simulink subsystem "VehicleDynamicsRing_subsysref"  (R2020a)
settings: Solver=VariableStepAuto  StartTime=0.0  StopTime=10.0  RelTol=1e-3
undefined symbols (not defined in the file): DRIVE_MODE, VDR
settings Model: Creator=Kiera  LastModifiedBy=Kiera

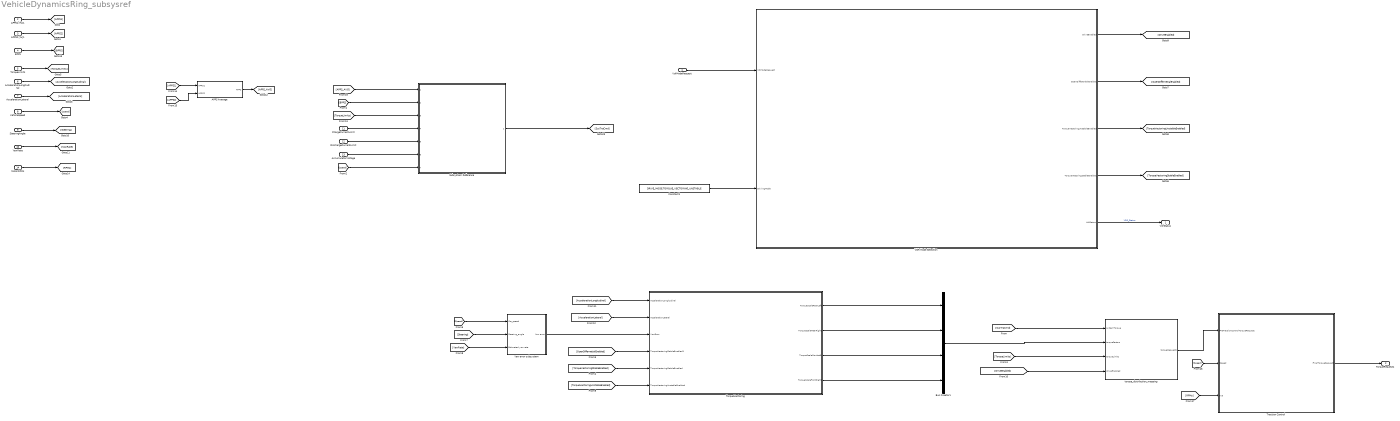
== system VehicleDynamicsRing_subsysref ==
  VdrModeRequest : Inport  OutDataTypeStr=Enum: MSR_REQUEST
  APPS1 [%]1 : Inport  Port=2  OutDataTypeStr=double
  APPS2 [%]1 : Inport  Port=3  OutDataTypeStr=double
  BPPS : Inport  Port=4  OutDataTypeStr=double
  TorqueLimits : Inport  Port=5  OutDataTypeStr=Bus: TorqueLimits
  AccelerationLongitudinal : Inport  Port=6  OutDataTypeStr=double
  AccelerationLateral : Inport  Port=7  OutDataTypeStr=double
  VehicleSpeed : Inport  Port=8
  SteeringAngle : Inport  Port=9
  YawRate : Inport  Port=10
  ChargeCurrentLimit : Inport  Port=11  OutDataTypeStr=double
  DischargeCurrentLimit : Inport  Port=12  OutDataTypeStr=double
  AccumulatorVoltage : Inport  Port=13
  MotorRPMs : Inport  Port=14  OutDataTypeStr=Bus: MotorRPMs
  APPS Average : Subsystem
  Bus Creator1 : BusCreator  Inputs=4
  Constant1 : Constant  Value=DRIVE_MODE.TORQUE_VECTORING_UNSTABLE
  Subsystem Reference : Subsystem  ReferencedSubsystem=PedalMapping_subsysref
  TorqueVectoring : Subsystem
  Traction Control : Subsystem
  VDR Mode Selection : Stateflow chart  TreatAsAtomicUnit=on
  Yaw error subsystem : Subsystem
  torque_distribution_mapping : MATLAB Function  TreatAsAtomicUnit=on
  VdrStatus : Outport  OutDataTypeStr=Enum: RING_STATUS  VectorParamsAs1DForOutWhenUnconnected=off
  TorqueRequests : Outport  Port=2  OutDataTypeStr=Bus: TorqueRequests  VectorParamsAs1DForOutWhenUnconnected=off
  wires:
  Yaw error subsystem/1(Yaw error) -> TorqueVectoring/3(YawError)
  YawRate/1 -> [YawRate]
  APPS2 [%]1/1 -> [APPS2]
  APPS1 [%]1/1 -> [APPS1]
  Bus Creator1/1 -> torque_distribution_mapping/2(torqueFactors)
  [OpenDiffernetialEnabled] -> TorqueVectoring/4(TorqueVectoringStableEnabled1)
  [Speed] -> Traction Control/2(Speed)
  MotorRPMs/1 -> [RPMs]
  TorqueVectoring/4(TorqueScaleFrontRight) -> Bus Creator1/4
  [RPMs] -> Traction Control/3(In3)
  Traction Control/1(FinalTorqueRequest) -> TorqueRequests/1
  VDR Mode Selection/3(TorqueVectoringUnstableEnabled) -> [TorqueVectoringUnstableEnabled]
  TorqueVectoring/3(TorqueScaleFrontLeft) -> Bus Creator1/3
  AccumulatorVoltage/1 -> Subsystem Reference/6
  [APPS2] -> APPS Average/2(APPS2)
  torque_distribution_mapping/1(torqueRequests) -> Traction Control/1(PreTractionControlTorqueRequest)
  VdrModeRequest/1 -> VDR Mode Selection/1(VdrModeRequest)
  DischargeCurrentLimit/1 -> Subsystem Reference/5
  BPPS/1 -> [BPPS]
  APPS Average/1(APPS) -> [APPS_AVG]
  VehicleSpeed/1 -> [Speed]
  Subsystem Reference/1 -> [SysTrqCmd]
  [SysTrqCmd] -> torque_distribution_mapping/1(systemTorque)
  AccelerationLongitudinal/1 -> [AccelerationLongitudinal]
  [APPS_AVG] -> Subsystem Reference/1
  [APPS1] -> APPS Average/1(APPS1)
  [Speed] -> Yaw error subsystem/1(Car_speed)
  TorqueVectoring/1(TorqueScaleRearLeft) -> Bus Creator1/1
  [YawRate] -> Yaw error subsystem/3("Estimated yaw rate ")
  [TorqueLimits] -> torque_distribution_mapping/3(torqueLimits)
  SteeringAngle/1 -> [Steering]
  Constant1/1 -> VDR Mode Selection/2(DrivingMode)
  [DriveEnabled] -> torque_distribution_mapping/4(driveEnabled)
  [AccelerationLongitudinal] -> TorqueVectoring/1("AccelerationLongitudinal ")
  VDR Mode Selection/1(DriveEnabled) -> [DriveEnabled]
  AccelerationLateral/1 -> [AccelerationLateral]
  VDR Mode Selection/5(VdrStatus) -> VdrStatus/1  "VDR_Status"
  [TorqueVectoringUnstableEnabled] -> TorqueVectoring/6(TorqueVectoringUnstableEnabled)
  [TorqueLimits] -> Subsystem Reference/3
  [BPPS] -> Subsystem Reference/2
  VDR Mode Selection/2(OpenDifferentialEnabled) -> [OpenDiffernetialEnabled]
  TorqueLimits/1 -> [TorqueLimits]
  [TorqueVectoringStableEnabled] -> TorqueVectoring/5(TorqueVectoringStableEnabled)
  [Steering] -> Yaw error subsystem/2(Steering_angle)
  ChargeCurrentLimit/1 -> Subsystem Reference/4
  [Speed] -> Subsystem Reference/7
  VDR Mode Selection/4(TorqueVectoringStableEnabled) -> [TorqueVectoringStableEnabled]
  [AccelerationLateral] -> TorqueVectoring/2(AccelerationLateral)
  TorqueVectoring/2(TorqueScaleRearRight) -> Bus Creator1/2

== system VehicleDynamicsRing_subsysref/APPS Average ==
  APPS1 : Inport
  APPS2 : Inport  Port=2
  Add : Sum
  Constant : Constant  Value=2
  Divide : Product  Inputs=*/
  APPS : Outport  VectorParamsAs1DForOutWhenUnconnected=off
  wires:
  Divide/1 -> APPS/1
  APPS2/1 -> Add/2
  APPS1/1 -> Add/1
  Add/1 -> Divide/1
  Constant/1 -> Divide/2

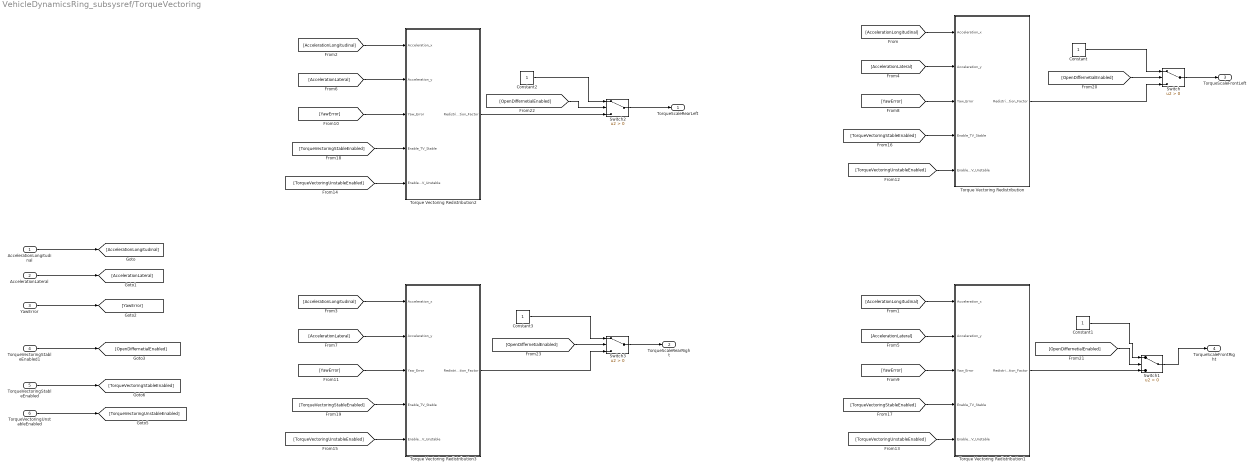
== system VehicleDynamicsRing_subsysref/TorqueVectoring ==
  "AccelerationLongitudinal " : Inport
  AccelerationLateral : Inport  Port=2
  YawError : Inport  Port=3
  TorqueVectoringStableEnabled1 : Inport  Port=4
  TorqueVectoringStableEnabled : Inport  Port=5
  TorqueVectoringUnstableEnabled : Inport  Port=6
  Constant{,1..3} (4 alike) : Constant
  Switch{,1..3} (4 alike) : Switch  Criteria=u2 > Threshold
  Torque Vectoring Redistribution : Subsystem  AncestorBlock=TorqueVectoringAlgorithmLib/Torque Vectoring Redistribution  mask{wheel_1=Front, wheel_2=Left}
      mask prompts: wheel_1 "Front or Rear Wheel"; wheel_2 "Left or Right Wheel"
      mask init:
      | %Front vs Rear Modifier
      | if(wheel_1 == 1) %Front Wheel
      |     stable_longitudinal_mod = -1;
      | else %Rear Wheel
      |     stable_longitudinal_mod = 1;
      | end
      | 
      | %Left vs Rear Modifier
      | if(wheel_2 == 1) %Left Wheel
      |     unstable_mod = -1;
      |     stable_lateral_mod = -1;
      | else %Right Wheel
      |     unstable_mod = 1;
      |     stable_lateral_mod = 1;
      | end
      mask TypeOptions wheel_1: Front | Rear
      mask TypeOptions wheel_2: Left | Right
      mask DialogControl DescGroupVar Prompt: Torque Vectoring Configurations
      mask DialogControl DescTextVar Prompt: Select the wheel for the torque vectoring configuration.
  Torque Vectoring Redistribution1 : Subsystem  AncestorBlock=TorqueVectoringAlgorithmLib/Torque Vectoring Redistribution  mask{wheel_1=Front, wheel_2=Right}
      mask prompts: wheel_1 "Front or Rear Wheel"; wheel_2 "Left or Right Wheel"
      mask init: same as VehicleDynamicsRing_subsysref/TorqueVectoring/Torque Vectoring Redistribution
      mask TypeOptions wheel_1: Front | Rear
      mask TypeOptions wheel_2: Left | Right
      mask DialogControl DescGroupVar Prompt: Torque Vectoring Configurations
      mask DialogControl DescTextVar Prompt: Select the wheel for the torque vectoring configuration.
  Torque Vectoring Redistribution2 : Subsystem  AncestorBlock=TorqueVectoringAlgorithmLib/Torque Vectoring Redistribution  mask{wheel_1=Rear, wheel_2=Left}
      mask prompts: wheel_1 "Front or Rear Wheel"; wheel_2 "Left or Right Wheel"
      mask init: same as VehicleDynamicsRing_subsysref/TorqueVectoring/Torque Vectoring Redistribution
      mask TypeOptions wheel_1: Front | Rear
      mask TypeOptions wheel_2: Left | Right
      mask DialogControl DescGroupVar Prompt: Torque Vectoring Configurations
      mask DialogControl DescTextVar Prompt: Select the wheel for the torque vectoring configuration.
  Torque Vectoring Redistribution3 : Subsystem  AncestorBlock=TorqueVectoringAlgorithmLib/Torque Vectoring Redistribution  mask{wheel_1=Rear, wheel_2=Right}
      mask prompts: wheel_1 "Front or Rear Wheel"; wheel_2 "Left or Right Wheel"
      mask init: same as VehicleDynamicsRing_subsysref/TorqueVectoring/Torque Vectoring Redistribution
      mask TypeOptions wheel_1: Front | Rear
      mask TypeOptions wheel_2: Left | Right
      mask DialogControl DescGroupVar Prompt: Torque Vectoring Configurations
      mask DialogControl DescTextVar Prompt: Select the wheel for the torque vectoring configuration.
  TorqueScaleRearLeft : Outport  VectorParamsAs1DForOutWhenUnconnected=off
  TorqueScaleRearRight : Outport  Port=2  VectorParamsAs1DForOutWhenUnconnected=off
  TorqueScaleFrontLeft : Outport  Port=3  VectorParamsAs1DForOutWhenUnconnected=off
  TorqueScaleFrontRight : Outport  Port=4  VectorParamsAs1DForOutWhenUnconnected=off
  wires:
  "AccelerationLongitudinal "/1 -> [AccelerationLongitudinal]
  AccelerationLateral/1 -> [AccelerationLateral]
  YawError/1 -> [YawError]
  TorqueVectoringUnstableEnabled/1 -> [TorqueVectoringUnstableEnabled]
  [AccelerationLongitudinal] -> Torque Vectoring Redistribution2/1(Acceleration_x)
  [AccelerationLongitudinal] -> Torque Vectoring Redistribution3/1(Acceleration_x)
  [AccelerationLateral] -> Torque Vectoring Redistribution2/2(Acceleration_y)
  [AccelerationLateral] -> Torque Vectoring Redistribution3/2(Acceleration_y)
  [YawError] -> Torque Vectoring Redistribution2/3(Yaw_Error)
  [YawError] -> Torque Vectoring Redistribution3/3(Yaw_Error)
  TorqueVectoringStableEnabled/1 -> [TorqueVectoringStableEnabled]
  [TorqueVectoringUnstableEnabled] -> Torque Vectoring Redistribution2/5(Enable_TV_Unstable)
  [TorqueVectoringUnstableEnabled] -> Torque Vectoring Redistribution3/5(Enable_TV_Unstable)
  [TorqueVectoringStableEnabled] -> Torque Vectoring Redistribution2/4(Enable_TV_Stable)
  [TorqueVectoringStableEnabled] -> Torque Vectoring Redistribution3/4(Enable_TV_Stable)
  TorqueVectoringStableEnabled1/1 -> [OpenDiffernetialEnabled]
  [TorqueVectoringStableEnabled] -> Torque Vectoring Redistribution/4(Enable_TV_Stable)
  [TorqueVectoringUnstableEnabled] -> Torque Vectoring Redistribution/5(Enable_TV_Unstable)
  [YawError] -> Torque Vectoring Redistribution/3(Yaw_Error)
  [AccelerationLateral] -> Torque Vectoring Redistribution/2(Acceleration_y)
  [AccelerationLongitudinal] -> Torque Vectoring Redistribution/1(Acceleration_x)
  [TorqueVectoringStableEnabled] -> Torque Vectoring Redistribution1/4(Enable_TV_Stable)
  [YawError] -> Torque Vectoring Redistribution1/3(Yaw_Error)
  [AccelerationLongitudinal] -> Torque Vectoring Redistribution1/1(Acceleration_x)
  [TorqueVectoringUnstableEnabled] -> Torque Vectoring Redistribution1/5(Enable_TV_Unstable)
  [AccelerationLateral] -> Torque Vectoring Redistribution1/2(Acceleration_y)
  [OpenDiffernetialEnabled] -> Switch/2
  Switch/1 -> TorqueScaleFrontLeft/1
  [OpenDiffernetialEnabled] -> Switch1/2
  Switch1/1 -> TorqueScaleFrontRight/1
  Constant1/1 -> Switch1/1
  Torque Vectoring Redistribution1/1(Redistribution_Factor) -> Switch1/3
  Torque Vectoring Redistribution/1(Redistribution_Factor) -> Switch/3
  Constant/1 -> Switch/1
  Constant2/1 -> Switch2/1
  [OpenDiffernetialEnabled] -> Switch2/2
  Switch2/1 -> TorqueScaleRearLeft/1
  Torque Vectoring Redistribution2/1(Redistribution_Factor) -> Switch2/3
  Constant3/1 -> Switch3/1
  [OpenDiffernetialEnabled] -> Switch3/2
  Switch3/1 -> TorqueScaleRearRight/1
  Torque Vectoring Redistribution3/1(Redistribution_Factor) -> Switch3/3

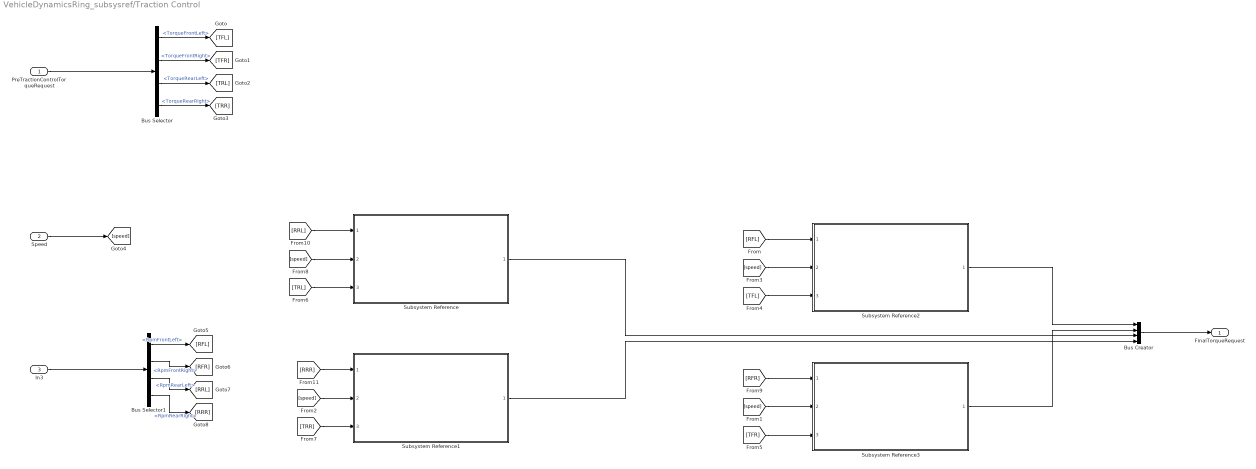
== system VehicleDynamicsRing_subsysref/Traction Control ==
  PreTractionControlTorqueRequest : Inport
  Speed : Inport  Port=2
  In3 : Inport  Port=3
  Bus Creator : BusCreator  Inputs=4  OutDataTypeStr=Bus: TorqueRequests
  Bus Selector : BusSelector  OutputSignals=TorqueFrontLeft,TorqueFrontRight,TorqueRearLeft,TorqueRearRight
  Bus Selector1 : BusSelector  OutputSignals=RpmFrontLeft,RpmFrontRight,RpmRearLeft,RpmRearRight
  Subsystem Reference{,1..3} (4 alike) : Subsystem  ReferencedSubsystem=TractionControl_subsysref
  FinalTorqueRequest : Outport  VectorParamsAs1DForOutWhenUnconnected=off
  wires:
  Subsystem Reference1/1 -> Bus Creator/4
  Subsystem Reference/1 -> Bus Creator/3
  Subsystem Reference3/1 -> Bus Creator/2
  Subsystem Reference2/1 -> Bus Creator/1
  Bus Creator/1 -> FinalTorqueRequest/1
  [RFR] -> Subsystem Reference3/1
  [RFL] -> Subsystem Reference2/1
  [RRL] -> Subsystem Reference/1
  [RRR] -> Subsystem Reference1/1
  Bus Selector1/4 -> [RRR]  "<RpmRearRight>"
  Bus Selector1/3 -> [RRL]  "<RpmRearLeft>"
  Bus Selector1/2 -> [RFR]  "<RpmFrontRight>"
  Bus Selector1/1 -> [RFL]  "<RpmFrontLeft>"
  [speed] -> Subsystem Reference3/2
  [speed] -> Subsystem Reference1/2
  [speed] -> Subsystem Reference2/2
  [speed] -> Subsystem Reference/2
  [TRR] -> Subsystem Reference1/3
  [TRL] -> Subsystem Reference/3
  [TFR] -> Subsystem Reference3/3
  [TFL] -> Subsystem Reference2/3
  In3/1 -> Bus Selector1/1
  Speed/1 -> [speed]
  Bus Selector/4 -> [TRR]  "<TorqueRearRight>"
  Bus Selector/3 -> [TRL]  "<TorqueRearLeft>"
  Bus Selector/2 -> [TFR]  "<TorqueFrontRight>"
  Bus Selector/1 -> [TFL]  "<TorqueFrontLeft>"
  PreTractionControlTorqueRequest/1 -> Bus Selector/1

== system VehicleDynamicsRing_subsysref/Yaw error subsystem ==
  Car_speed : Inport
  Steering_angle : Inport  Port=2
  "Estimated yaw rate " : Inport  Port=3
  Desired yaw rate calculation : Subsystem
  Subtract : Sum  Inputs=+-
  Yaw rate estimatior : Subsystem  Commented=on
  Yaw error : Outport  VectorParamsAs1DForOutWhenUnconnected=off
  wires:
  Steering_angle/1 -> Desired yaw rate calculation/2(Steering angle)
  Subtract/1 -> Yaw error/1
  "Estimated yaw rate "/1 -> Subtract/2
  Car_speed/1 -> Desired yaw rate calculation/1(Car speed)
  Desired yaw rate calculation/1(Desired yaw rate) -> Subtract/1

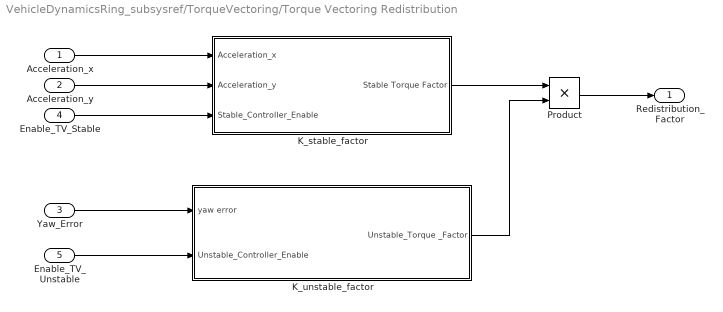
== system VehicleDynamicsRing_subsysref/TorqueVectoring/Torque Vectoring Redistribution ==
  Acceleration_x : Inport
  Acceleration_y : Inport  Port=2
  Yaw_Error : Inport  Port=3
  Enable_TV_Stable : Inport  Port=4
  Enable_TV_Unstable : Inport  Port=5
  K_stable_factor : Subsystem
  K_unstable_factor : Subsystem
  Product : Product
  Redistribution_Factor : Outport  VectorParamsAs1DForOutWhenUnconnected=off
  wires:
  Enable_TV_Unstable/1 -> K_unstable_factor/2(Unstable_Controller_Enable)
  Enable_TV_Stable/1 -> K_stable_factor/3(Stable_Controller_Enable)
  Product/1 -> Redistribution_Factor/1
  Acceleration_y/1 -> K_stable_factor/2(Acceleration_y)
  Yaw_Error/1 -> K_unstable_factor/1(yaw error)
  Acceleration_x/1 -> K_stable_factor/1(Acceleration_x)
  K_stable_factor/1(Stable Torque Factor) -> Product/1
  K_unstable_factor/1(Unstable_Torque _Factor) -> Product/2

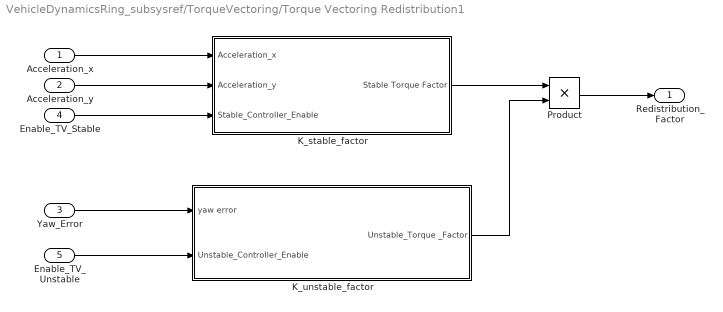
== system VehicleDynamicsRing_subsysref/TorqueVectoring/Torque Vectoring Redistribution1 ==
  Acceleration_x : Inport
  Acceleration_y : Inport  Port=2
  Yaw_Error : Inport  Port=3
  Enable_TV_Stable : Inport  Port=4
  Enable_TV_Unstable : Inport  Port=5
  K_stable_factor : Subsystem
  K_unstable_factor : Subsystem
  Product : Product
  Redistribution_Factor : Outport  VectorParamsAs1DForOutWhenUnconnected=off
  wires:
  Enable_TV_Unstable/1 -> K_unstable_factor/2(Unstable_Controller_Enable)
  Enable_TV_Stable/1 -> K_stable_factor/3(Stable_Controller_Enable)
  Product/1 -> Redistribution_Factor/1
  Acceleration_y/1 -> K_stable_factor/2(Acceleration_y)
  Yaw_Error/1 -> K_unstable_factor/1(yaw error)
  Acceleration_x/1 -> K_stable_factor/1(Acceleration_x)
  K_stable_factor/1(Stable Torque Factor) -> Product/1
  K_unstable_factor/1(Unstable_Torque _Factor) -> Product/2

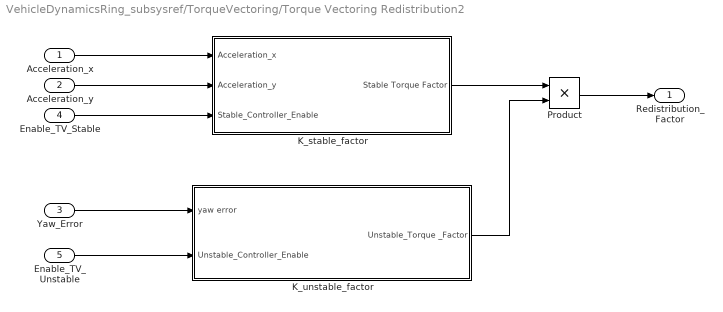
== system VehicleDynamicsRing_subsysref/TorqueVectoring/Torque Vectoring Redistribution2 ==
  Acceleration_x : Inport
  Acceleration_y : Inport  Port=2
  Yaw_Error : Inport  Port=3
  Enable_TV_Stable : Inport  Port=4
  Enable_TV_Unstable : Inport  Port=5
  K_stable_factor : Subsystem
  K_unstable_factor : Subsystem
  Product : Product
  Redistribution_Factor : Outport  VectorParamsAs1DForOutWhenUnconnected=off
  wires:
  Enable_TV_Unstable/1 -> K_unstable_factor/2(Unstable_Controller_Enable)
  Enable_TV_Stable/1 -> K_stable_factor/3(Stable_Controller_Enable)
  Product/1 -> Redistribution_Factor/1
  Acceleration_y/1 -> K_stable_factor/2(Acceleration_y)
  Yaw_Error/1 -> K_unstable_factor/1(yaw error)
  Acceleration_x/1 -> K_stable_factor/1(Acceleration_x)
  K_stable_factor/1(Stable Torque Factor) -> Product/1
  K_unstable_factor/1(Unstable_Torque _Factor) -> Product/2

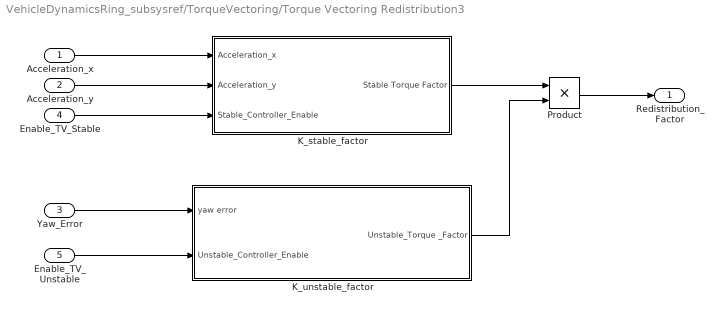
== system VehicleDynamicsRing_subsysref/TorqueVectoring/Torque Vectoring Redistribution3 ==
  Acceleration_x : Inport
  Acceleration_y : Inport  Port=2
  Yaw_Error : Inport  Port=3
  Enable_TV_Stable : Inport  Port=4
  Enable_TV_Unstable : Inport  Port=5
  K_stable_factor : Subsystem
  K_unstable_factor : Subsystem
  Product : Product
  Redistribution_Factor : Outport  VectorParamsAs1DForOutWhenUnconnected=off
  wires:
  Enable_TV_Unstable/1 -> K_unstable_factor/2(Unstable_Controller_Enable)
  Enable_TV_Stable/1 -> K_stable_factor/3(Stable_Controller_Enable)
  Product/1 -> Redistribution_Factor/1
  Acceleration_y/1 -> K_stable_factor/2(Acceleration_y)
  Yaw_Error/1 -> K_unstable_factor/1(yaw error)
  Acceleration_x/1 -> K_stable_factor/1(Acceleration_x)
  K_stable_factor/1(Stable Torque Factor) -> Product/1
  K_unstable_factor/1(Unstable_Torque _Factor) -> Product/2

== system VehicleDynamicsRing_subsysref/Yaw error subsystem/Desired yaw rate calculation ==
  Car speed : Inport
  Steering angle : Inport  Port=2
  Add : Sum
  "CM to front axel " : Constant  Value=VDR.l_f
  CM to rear axel : Constant  Value=VDR.l_r
  Divide : Product  Inputs=*/
  Product : Product
  Desired yaw rate : Outport  VectorParamsAs1DForOutWhenUnconnected=off
  wires:
  Steering angle/1 -> Product/2
  Add/1 -> Divide/2
  Divide/1 -> Desired yaw rate/1
  Car speed/1 -> Product/1
  Product/1 -> Divide/1
  CM to rear axel/1 -> Add/2
  "CM to front axel "/1 -> Add/1

== system VehicleDynamicsRing_subsysref/Yaw error subsystem/Yaw rate estimatior ==
  velocity-x : Inport
  steering angle : Inport  Port=2
  Divide : Product  Inputs=*/
  Product : Product
  Trigonometric Function : Trigonometry  Operator=tan
  Wheelbase : Constant  Value=VDR.l
  yaw rate estimate : Outport  VectorParamsAs1DForOutWhenUnconnected=off
  wires:
  steering angle/1 -> Trigonometric Function/1
  velocity-x/1 -> Product/1
  Trigonometric Function/1 -> Product/2
  Product/1 -> Divide/1
  Wheelbase/1 -> Divide/2
  Divide/1 -> yaw rate estimate/1

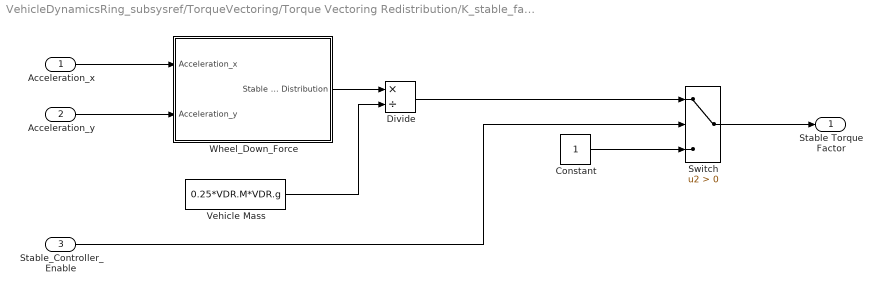
== system VehicleDynamicsRing_subsysref/TorqueVectoring/Torque Vectoring Redistribution/K_stable_factor ==
  Acceleration_x : Inport
  Acceleration_y : Inport  Port=2
  Stable_Controller_Enable : Inport  Port=3
  Constant : Constant
  Divide : Product  Inputs=*/
  Switch : Switch  Criteria=u2 > Threshold
  Vehicle Mass : Constant  Value=0.25*VDR.M*VDR.g
  Wheel_Down_Force : Subsystem
  Stable Torque Factor : Outport  VectorParamsAs1DForOutWhenUnconnected=off
  wires:
  Constant/1 -> Switch/3
  Switch/1 -> Stable Torque Factor/1
  Divide/1 -> Switch/1
  Stable_Controller_Enable/1 -> Switch/2
  Vehicle Mass/1 -> Divide/2
  Wheel_Down_Force/1(Stable Weigth Distribution) -> Divide/1
  Acceleration_x/1 -> Wheel_Down_Force/1(Acceleration_x)
  Acceleration_y/1 -> Wheel_Down_Force/2(Acceleration_y)

== system VehicleDynamicsRing_subsysref/TorqueVectoring/Torque Vectoring Redistribution/K_unstable_factor ==
  yaw error : Inport
  Unstable_Controller_Enable : Inport  Port=2
  Add : Sum
  Constant : Constant
  Constant1 : Constant
  Switch : Switch  Criteria=u2 > Threshold
  Unstable_Controller_Gain : Gain  Gain=VDR.Kp
  Unstable_Modifier : Gain  Gain=unstable_mod
  Unstable_Torque _Factor : Outport  VectorParamsAs1DForOutWhenUnconnected=off
  wires:
  Constant1/1 -> Switch/3
  Unstable_Controller_Enable/1 -> Switch/2
  Switch/1 -> Unstable_Torque _Factor/1
  Add/1 -> Switch/1
  Unstable_Modifier/1 -> Add/1
  yaw error/1 -> Unstable_Controller_Gain/1
  Constant/1 -> Add/2
  Unstable_Controller_Gain/1 -> Unstable_Modifier/1

== system VehicleDynamicsRing_subsysref/TorqueVectoring/Torque Vectoring Redistribution1/K_stable_factor ==
  Acceleration_x : Inport
  Acceleration_y : Inport  Port=2
  Stable_Controller_Enable : Inport  Port=3
  Constant : Constant
  Divide : Product  Inputs=*/
  Switch : Switch  Criteria=u2 > Threshold
  Vehicle Mass : Constant  Value=0.25*VDR.M*VDR.g
  Wheel_Down_Force : Subsystem
  Stable Torque Factor : Outport  VectorParamsAs1DForOutWhenUnconnected=off
  wires:
  Constant/1 -> Switch/3
  Switch/1 -> Stable Torque Factor/1
  Divide/1 -> Switch/1
  Stable_Controller_Enable/1 -> Switch/2
  Vehicle Mass/1 -> Divide/2
  Wheel_Down_Force/1(Stable Weigth Distribution) -> Divide/1
  Acceleration_x/1 -> Wheel_Down_Force/1(Acceleration_x)
  Acceleration_y/1 -> Wheel_Down_Force/2(Acceleration_y)

== system VehicleDynamicsRing_subsysref/TorqueVectoring/Torque Vectoring Redistribution1/K_unstable_factor ==
  yaw error : Inport
  Unstable_Controller_Enable : Inport  Port=2
  Add : Sum
  Constant : Constant
  Constant1 : Constant
  Switch : Switch  Criteria=u2 > Threshold
  Unstable_Controller_Gain : Gain  Gain=VDR.Kp
  Unstable_Modifier : Gain  Gain=unstable_mod
  Unstable_Torque _Factor : Outport  VectorParamsAs1DForOutWhenUnconnected=off
  wires:
  Constant1/1 -> Switch/3
  Unstable_Controller_Enable/1 -> Switch/2
  Switch/1 -> Unstable_Torque _Factor/1
  Add/1 -> Switch/1
  Unstable_Modifier/1 -> Add/1
  yaw error/1 -> Unstable_Controller_Gain/1
  Constant/1 -> Add/2
  Unstable_Controller_Gain/1 -> Unstable_Modifier/1

== system VehicleDynamicsRing_subsysref/TorqueVectoring/Torque Vectoring Redistribution2/K_stable_factor ==
  Acceleration_x : Inport
  Acceleration_y : Inport  Port=2
  Stable_Controller_Enable : Inport  Port=3
  Constant : Constant
  Divide : Product  Inputs=*/
  Switch : Switch  Criteria=u2 > Threshold
  Vehicle Mass : Constant  Value=0.25*VDR.M*VDR.g
  Wheel_Down_Force : Subsystem
  Stable Torque Factor : Outport  VectorParamsAs1DForOutWhenUnconnected=off
  wires:
  Constant/1 -> Switch/3
  Switch/1 -> Stable Torque Factor/1
  Divide/1 -> Switch/1
  Stable_Controller_Enable/1 -> Switch/2
  Vehicle Mass/1 -> Divide/2
  Wheel_Down_Force/1(Stable Weigth Distribution) -> Divide/1
  Acceleration_x/1 -> Wheel_Down_Force/1(Acceleration_x)
  Acceleration_y/1 -> Wheel_Down_Force/2(Acceleration_y)

== system VehicleDynamicsRing_subsysref/TorqueVectoring/Torque Vectoring Redistribution2/K_unstable_factor ==
  yaw error : Inport
  Unstable_Controller_Enable : Inport  Port=2
  Add : Sum
  Constant : Constant
  Constant1 : Constant
  Switch : Switch  Criteria=u2 > Threshold
  Unstable_Controller_Gain : Gain  Gain=VDR.Kp
  Unstable_Modifier : Gain  Gain=unstable_mod
  Unstable_Torque _Factor : Outport  VectorParamsAs1DForOutWhenUnconnected=off
  wires:
  Constant1/1 -> Switch/3
  Unstable_Controller_Enable/1 -> Switch/2
  Switch/1 -> Unstable_Torque _Factor/1
  Add/1 -> Switch/1
  Unstable_Modifier/1 -> Add/1
  yaw error/1 -> Unstable_Controller_Gain/1
  Constant/1 -> Add/2
  Unstable_Controller_Gain/1 -> Unstable_Modifier/1

== system VehicleDynamicsRing_subsysref/TorqueVectoring/Torque Vectoring Redistribution3/K_stable_factor ==
  Acceleration_x : Inport
  Acceleration_y : Inport  Port=2
  Stable_Controller_Enable : Inport  Port=3
  Constant : Constant
  Divide : Product  Inputs=*/
  Switch : Switch  Criteria=u2 > Threshold
  Vehicle Mass : Constant  Value=0.25*VDR.M*VDR.g
  Wheel_Down_Force : Subsystem
  Stable Torque Factor : Outport  VectorParamsAs1DForOutWhenUnconnected=off
  wires:
  Constant/1 -> Switch/3
  Switch/1 -> Stable Torque Factor/1
  Divide/1 -> Switch/1
  Stable_Controller_Enable/1 -> Switch/2
  Vehicle Mass/1 -> Divide/2
  Wheel_Down_Force/1(Stable Weigth Distribution) -> Divide/1
  Acceleration_x/1 -> Wheel_Down_Force/1(Acceleration_x)
  Acceleration_y/1 -> Wheel_Down_Force/2(Acceleration_y)

== system VehicleDynamicsRing_subsysref/TorqueVectoring/Torque Vectoring Redistribution3/K_unstable_factor ==
  yaw error : Inport
  Unstable_Controller_Enable : Inport  Port=2
  Add : Sum
  Constant : Constant
  Constant1 : Constant
  Switch : Switch  Criteria=u2 > Threshold
  Unstable_Controller_Gain : Gain  Gain=VDR.Kp
  Unstable_Modifier : Gain  Gain=unstable_mod
  Unstable_Torque _Factor : Outport  VectorParamsAs1DForOutWhenUnconnected=off
  wires:
  Constant1/1 -> Switch/3
  Unstable_Controller_Enable/1 -> Switch/2
  Switch/1 -> Unstable_Torque _Factor/1
  Add/1 -> Switch/1
  Unstable_Modifier/1 -> Add/1
  yaw error/1 -> Unstable_Controller_Gain/1
  Constant/1 -> Add/2
  Unstable_Controller_Gain/1 -> Unstable_Modifier/1

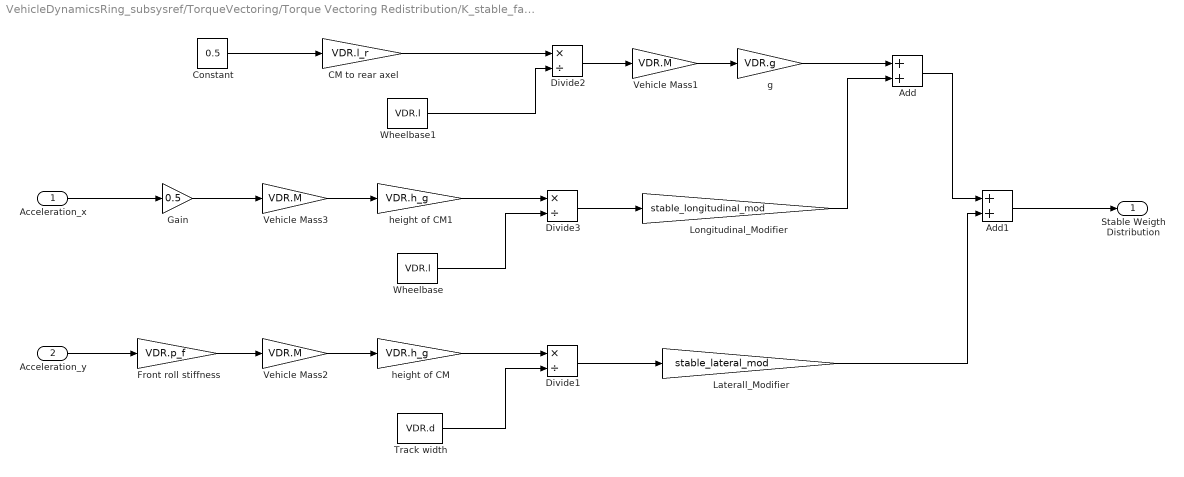
== system VehicleDynamicsRing_subsysref/TorqueVectoring/Torque Vectoring Redistribution/K_stable_factor/Wheel_Down_Force ==
  Acceleration_x : Inport
  Acceleration_y : Inport  Port=2
  Add : Sum
  Add1 : Sum
  CM to rear axel : Gain  Gain=VDR.l_r
  Constant : Constant  Value=0.5
  Divide1 : Product  Inputs=*/
  Divide2 : Product  Inputs=*/
  Divide3 : Product  Inputs=*/
  Front roll stiffness : Gain  Gain=VDR.p_f
  Gain : Gain  Gain=0.5
  Laterall_Modifier : Gain  Gain=stable_lateral_mod
  Longitudinal_Modifier : Gain  Gain=stable_longitudinal_mod
  Track width : Constant  Value=VDR.d
  Vehicle Mass1 : Gain  Gain=VDR.M
  Vehicle Mass2 : Gain  Gain=VDR.M
  Vehicle Mass3 : Gain  Gain=VDR.M
  Wheelbase : Constant  Value=VDR.l
  Wheelbase1 : Constant  Value=VDR.l
  g : Gain  Gain=VDR.g
  height of CM : Gain  Gain=VDR.h_g
  height of CM1 : Gain  Gain=VDR.h_g
  Stable Weigth Distribution : Outport  VectorParamsAs1DForOutWhenUnconnected=off
  wires:
  Gain/1 -> Vehicle Mass3/1
  Laterall_Modifier/1 -> Add1/2
  Add/1 -> Add1/1
  Longitudinal_Modifier/1 -> Add/2
  g/1 -> Add/1
  Track width/1 -> Divide1/2
  Wheelbase/1 -> Divide3/2
  Divide1/1 -> Laterall_Modifier/1
  Divide3/1 -> Longitudinal_Modifier/1
  Wheelbase1/1 -> Divide2/2
  Divide2/1 -> Vehicle Mass1/1
  Acceleration_y/1 -> Front roll stiffness/1
  Constant/1 -> CM to rear axel/1
  CM to rear axel/1 -> Divide2/1
  Acceleration_x/1 -> Gain/1
  Front roll stiffness/1 -> Vehicle Mass2/1
  Vehicle Mass1/1 -> g/1
  Vehicle Mass2/1 -> height of CM/1
  height of CM/1 -> Divide1/1
  Vehicle Mass3/1 -> height of CM1/1
  height of CM1/1 -> Divide3/1
  Add1/1 -> Stable Weigth Distribution/1

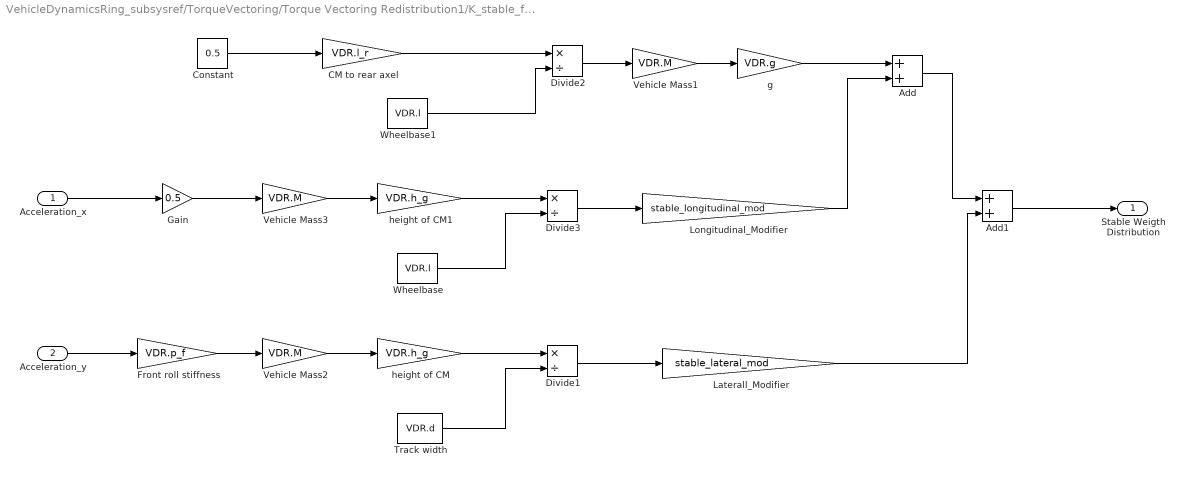
== system VehicleDynamicsRing_subsysref/TorqueVectoring/Torque Vectoring Redistribution1/K_stable_factor/Wheel_Down_Force ==
  Acceleration_x : Inport
  Acceleration_y : Inport  Port=2
  Add : Sum
  Add1 : Sum
  CM to rear axel : Gain  Gain=VDR.l_r
  Constant : Constant  Value=0.5
  Divide1 : Product  Inputs=*/
  Divide2 : Product  Inputs=*/
  Divide3 : Product  Inputs=*/
  Front roll stiffness : Gain  Gain=VDR.p_f
  Gain : Gain  Gain=0.5
  Laterall_Modifier : Gain  Gain=stable_lateral_mod
  Longitudinal_Modifier : Gain  Gain=stable_longitudinal_mod
  Track width : Constant  Value=VDR.d
  Vehicle Mass1 : Gain  Gain=VDR.M
  Vehicle Mass2 : Gain  Gain=VDR.M
  Vehicle Mass3 : Gain  Gain=VDR.M
  Wheelbase : Constant  Value=VDR.l
  Wheelbase1 : Constant  Value=VDR.l
  g : Gain  Gain=VDR.g
  height of CM : Gain  Gain=VDR.h_g
  height of CM1 : Gain  Gain=VDR.h_g
  Stable Weigth Distribution : Outport  VectorParamsAs1DForOutWhenUnconnected=off
  wires:
  Gain/1 -> Vehicle Mass3/1
  Laterall_Modifier/1 -> Add1/2
  Add/1 -> Add1/1
  Longitudinal_Modifier/1 -> Add/2
  g/1 -> Add/1
  Track width/1 -> Divide1/2
  Wheelbase/1 -> Divide3/2
  Divide1/1 -> Laterall_Modifier/1
  Divide3/1 -> Longitudinal_Modifier/1
  Wheelbase1/1 -> Divide2/2
  Divide2/1 -> Vehicle Mass1/1
  Acceleration_y/1 -> Front roll stiffness/1
  Constant/1 -> CM to rear axel/1
  CM to rear axel/1 -> Divide2/1
  Acceleration_x/1 -> Gain/1
  Front roll stiffness/1 -> Vehicle Mass2/1
  Vehicle Mass1/1 -> g/1
  Vehicle Mass2/1 -> height of CM/1
  height of CM/1 -> Divide1/1
  Vehicle Mass3/1 -> height of CM1/1
  height of CM1/1 -> Divide3/1
  Add1/1 -> Stable Weigth Distribution/1

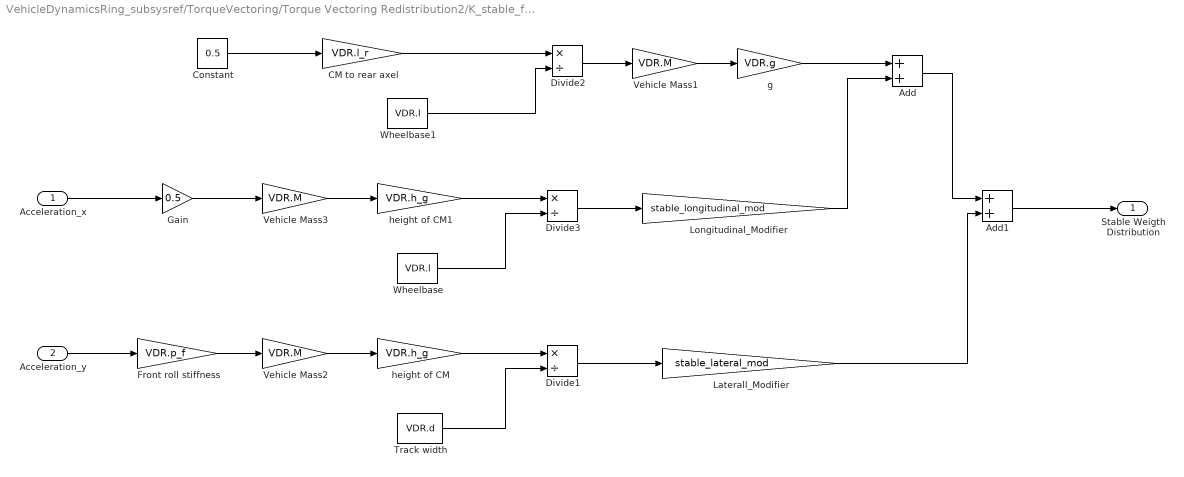
== system VehicleDynamicsRing_subsysref/TorqueVectoring/Torque Vectoring Redistribution2/K_stable_factor/Wheel_Down_Force ==
  Acceleration_x : Inport
  Acceleration_y : Inport  Port=2
  Add : Sum
  Add1 : Sum
  CM to rear axel : Gain  Gain=VDR.l_r
  Constant : Constant  Value=0.5
  Divide1 : Product  Inputs=*/
  Divide2 : Product  Inputs=*/
  Divide3 : Product  Inputs=*/
  Front roll stiffness : Gain  Gain=VDR.p_f
  Gain : Gain  Gain=0.5
  Laterall_Modifier : Gain  Gain=stable_lateral_mod
  Longitudinal_Modifier : Gain  Gain=stable_longitudinal_mod
  Track width : Constant  Value=VDR.d
  Vehicle Mass1 : Gain  Gain=VDR.M
  Vehicle Mass2 : Gain  Gain=VDR.M
  Vehicle Mass3 : Gain  Gain=VDR.M
  Wheelbase : Constant  Value=VDR.l
  Wheelbase1 : Constant  Value=VDR.l
  g : Gain  Gain=VDR.g
  height of CM : Gain  Gain=VDR.h_g
  height of CM1 : Gain  Gain=VDR.h_g
  Stable Weigth Distribution : Outport  VectorParamsAs1DForOutWhenUnconnected=off
  wires:
  Gain/1 -> Vehicle Mass3/1
  Laterall_Modifier/1 -> Add1/2
  Add/1 -> Add1/1
  Longitudinal_Modifier/1 -> Add/2
  g/1 -> Add/1
  Track width/1 -> Divide1/2
  Wheelbase/1 -> Divide3/2
  Divide1/1 -> Laterall_Modifier/1
  Divide3/1 -> Longitudinal_Modifier/1
  Wheelbase1/1 -> Divide2/2
  Divide2/1 -> Vehicle Mass1/1
  Acceleration_y/1 -> Front roll stiffness/1
  Constant/1 -> CM to rear axel/1
  CM to rear axel/1 -> Divide2/1
  Acceleration_x/1 -> Gain/1
  Front roll stiffness/1 -> Vehicle Mass2/1
  Vehicle Mass1/1 -> g/1
  Vehicle Mass2/1 -> height of CM/1
  height of CM/1 -> Divide1/1
  Vehicle Mass3/1 -> height of CM1/1
  height of CM1/1 -> Divide3/1
  Add1/1 -> Stable Weigth Distribution/1

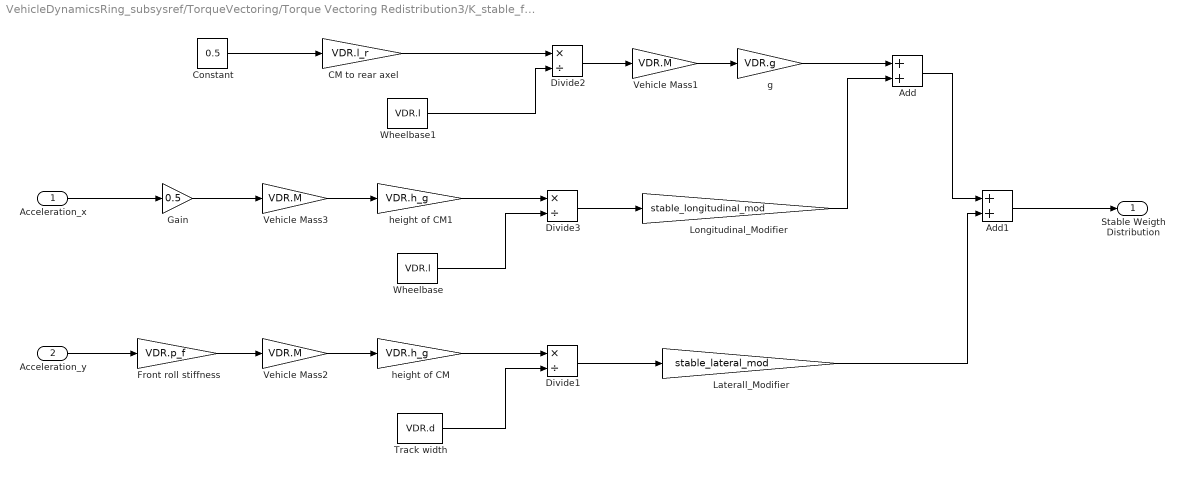
== system VehicleDynamicsRing_subsysref/TorqueVectoring/Torque Vectoring Redistribution3/K_stable_factor/Wheel_Down_Force ==
  Acceleration_x : Inport
  Acceleration_y : Inport  Port=2
  Add : Sum
  Add1 : Sum
  CM to rear axel : Gain  Gain=VDR.l_r
  Constant : Constant  Value=0.5
  Divide1 : Product  Inputs=*/
  Divide2 : Product  Inputs=*/
  Divide3 : Product  Inputs=*/
  Front roll stiffness : Gain  Gain=VDR.p_f
  Gain : Gain  Gain=0.5
  Laterall_Modifier : Gain  Gain=stable_lateral_mod
  Longitudinal_Modifier : Gain  Gain=stable_longitudinal_mod
  Track width : Constant  Value=VDR.d
  Vehicle Mass1 : Gain  Gain=VDR.M
  Vehicle Mass2 : Gain  Gain=VDR.M
  Vehicle Mass3 : Gain  Gain=VDR.M
  Wheelbase : Constant  Value=VDR.l
  Wheelbase1 : Constant  Value=VDR.l
  g : Gain  Gain=VDR.g
  height of CM : Gain  Gain=VDR.h_g
  height of CM1 : Gain  Gain=VDR.h_g
  Stable Weigth Distribution : Outport  VectorParamsAs1DForOutWhenUnconnected=off
  wires:
  Gain/1 -> Vehicle Mass3/1
  Laterall_Modifier/1 -> Add1/2
  Add/1 -> Add1/1
  Longitudinal_Modifier/1 -> Add/2
  g/1 -> Add/1
  Track width/1 -> Divide1/2
  Wheelbase/1 -> Divide3/2
  Divide1/1 -> Laterall_Modifier/1
  Divide3/1 -> Longitudinal_Modifier/1
  Wheelbase1/1 -> Divide2/2
  Divide2/1 -> Vehicle Mass1/1
  Acceleration_y/1 -> Front roll stiffness/1
  Constant/1 -> CM to rear axel/1
  CM to rear axel/1 -> Divide2/1
  Acceleration_x/1 -> Gain/1
  Front roll stiffness/1 -> Vehicle Mass2/1
  Vehicle Mass1/1 -> g/1
  Vehicle Mass2/1 -> height of CM/1
  height of CM/1 -> Divide1/1
  Vehicle Mass3/1 -> height of CM1/1
  height of CM1/1 -> Divide3/1
  Add1/1 -> Stable Weigth Distribution/1

== matlab function VehicleDynamicsRing_subsysref/torque_distribution_mapping ==
  data: systemTorque input; torqueFactors input size=4; torqueRequests output Bus: TorqueRequests; torqueLimits input Bus: TorqueLimits; driveEnabled input
function torqueRequests = torque_vectoring(systemTorque,torqueFactors,torqueLimits, driveEnabled)
% This function calculates the optimal torque distribution based on the
% relative torque scaling factors (determined by vehicle acceleration and
% understeering/oversteering) and the torque limits for each motor.
% torque_scales: fl, fr, rl, rr
% torque_limits: fl, fr, rl, rr

% Optimal torque distribution is determined by maintaining the relative
% torque scaling factors and using a nominal torque such that system torque
% is maximized and the torque limits for all motors are not exceeded

% Ex: Torque_fl = torque_scales[1]*torque_nominal

torqueRequests.TorqueFrontLeft = 0;
torqueRequests.TorqueFrontRight = 0;
torqueRequests.TorqueRearLeft = 0;
torqueRequests.TorqueRearRight = 0;
nominalTorque = systemTorque/4;
tempNominalTorque = [nominalTorque,nominalTorque,nominalTorque,nominalTorque];

if(driveEnabled)
    if(torqueFactors(1) ~= 0)
        tempNominalTorque(1) = torqueLimits.TorqueLimitFrontLeft/torqueFactors(1);
    end
    if(torqueFactors(2) ~= 0)
        tempNominalTorque(2) = torqueLimits.TorqueLimitFrontRight/torqueFactors(2);
    end
    if(torqueFactors(3) ~= 0)
        tempNominalTorque(3) = torqueLimits.TorqueLimitRearLeft/torqueFactors(3);
    end
    if(torqueFactors(4) ~= 0)
        tempNominalTorque(4) = torqueLimits.TorqueLimitRearRight/torqueFactors(4);
    end
    
    nominalTorque = min(tempNominalTorque);
  
    torqueRequests.TorqueFrontLeft = nominalTorque * torqueFactors(1);
    torqueRequests.TorqueFrontRight = nominalTorque * torqueFactors(2);
    torqueRequests.TorqueRearLeft = nominalTorque * torqueFactors(3);
    torqueRequests.TorqueRearRight = nominalTorque * torqueFactors(4);
    
end
end

% torque_requests = [0,0,0,0];
% torque_nominal = 0;
% total_system_torque = 0;
% temp_system_torque = 0;
% limit_fail = false;

% for i = 1:size(torque_scales)
%     limit_fail = false;
%     temp_system_torque = 0;
%     temp_nominal = torque_limits[i]/torque_scales[i];
%     for j = 1:size(torque_scales)
%         if(temp_nominal*torque_scales[j] > torque_limits[j])
%             limit_fail = true;
%             break;
%         end
%         temp_system_torque = temp_system_torque + temp_nominal*torque_scales[j];
%     end
%     if(limit_fail)
%         continue;
%     end
%     if(temp_system_torque > total_system_torque)
%         total_system_torque = temp_system_torque;
%         torque_nominal = temp_nominal;
%     end
% end
% 
% for i = 1:size(torque_scales)
%     torque_requests[i] = torque_nominal*torque_scales[i];
% end
% 
% end %done

== stateflow chart VehicleDynamicsRing_subsysref/VDR Mode Selection ==
  state OFF
    during:
    TorqueVectoringUnstableEnabled = false;
    DriveEnabled = false;
    TorqueVectoringStableEnabled = false;
    VdrStatus = RING_STATUS.OFF;
  state SHUTDOWN
    entry:
    VdrStatus = RING_STATUS.SHUTDOWN_IN_PROGRESS_HV;
    %TODO: Add checks for shutdown
    VdrStatus = RING_STATUS.SHUTDOWN_COMPLETE_HV;
  state OPERATIONAL
    state STARTUP
      entry:
      VdrStatus = RING_STATUS.STARTUP_IN_PROGRESS_HV;
    state RUNNING
      entry:
      DriveEnabled = true;
      VdrStatus = RING_STATUS.RUNNING;
      exit:
      DriveEnabled = false;
      state DRIVING_MODE
      state TORQUE_VECTORING
        state CHECK_TORQUE_VECTORING_MODE
        state TORQUE_VECTORING_UNSTABLE
          entry:
          TorqueVectoringUnstableEnabled = true;
          exit:
          TorqueVectoringUnstableEnabled = false;
        state TORQUE_VECTORING_STABLE
          entry:
          TorqueVectoringStableEnabled = true;
          exit:
          TorqueVectoringStableEnabled = false;
        (default) -> CHECK_TORQUE_VECTORING_MODE
        CHECK_TORQUE_VECTORING_MODE -> TORQUE_VECTORING_UNSTABLE [order 1] : [DrivingMode == DRIVE_MODE.TORQUE_VECTORING_STABLE]
        CHECK_TORQUE_VECTORING_MODE -> TORQUE_VECTORING_STABLE [order 2] : [DrivingMode == DRIVE_MODE.TORQUE_VECTORING_STABLE]
        TORQUE_VECTORING_UNSTABLE -> TORQUE_VECTORING_STABLE : [DrivingMode == DRIVE_MODE.TORQUE_VECTORING_STABLE]
      state TORQUE_VECTORING_STABLE1
        entry:
        OpenDifferentialEnabled = true;
        exit:
        OpenDifferentialEnabled = false;
      (default) -> DRIVING_MODE
      DRIVING_MODE -> TORQUE_VECTORING [order 1] : [DrivingMode == DRIVE_MODE.TORQUE_VECTORING_STABLE ||...
          | DrivingMode == DRIVE_MODE.TORQUE_VECTORING_STABLE]
      DRIVING_MODE -> TORQUE_VECTORING_STABLE1 [order 2] : [DrivingMode == DRIVE_MODE.OPEN_DIFFERENTIAL]
      TORQUE_VECTORING -> TORQUE_VECTORING_STABLE1 : [DrivingMode == DRIVE_MODE.OPEN_DIFFERENTIAL]
    state STARTUP_PASS
      entry:
      VdrStatus = RING_STATUS.STARTUP_COMPLETE_HV;
    (default) -> STARTUP
    STARTUP -> STARTUP_PASS
    STARTUP_PASS -> RUNNING : [VdrModeRequest == VDR.Mode.DRIVING &&...
        | VdrStatus == RING_STATUS.STARTUP_COMPLETE_HV]
  (default) -> OFF
  OPERATIONAL -> SHUTDOWN : [VdrModeRequest == MSR_REQUEST.SHUTDOWN_HV]
  OFF -> OPERATIONAL : [VdrModeRequest == MSR_REQUEST.STARTUP_HV]
  data: VdrModeRequest input Enum: MSR_REQUEST; VDR parameter; DriveEnabled output boolean; OpenDifferentialEnabled output boolean; TorqueVectoringUnstableEnabled output boolean; TorqueVectoringStableEnabled output boolean; VdrStatus output Enum: RING_STATUS; DrivingMode input Enum: DRIVE_MODE
  function StartUpTestCheck:
    | function StartUpTestCheck
    | 
    | aVarTruthTableCondition_1 = false;
    | aVarTruthTableCondition_2 = false;
    | aVarTruthTableCondition_3 = false;
    | aVarTruthTableCondition_4 = false;
    | 
    | 
    | % Look at APPS
    | 
    | aVarTruthTableCondition_1 = logical(APPS >= 0 && APPS <= 100);
    | 
    | % Car is not moving check: accel-x
    | 
    | aVarTruthTableCondition_2 = logical(abs(Accel_X) < VDR.MinAccelX);
    | 
    | % Car is not moving check: accel-y
    | 
    | aVarTruthTableCondition_3 = logical(abs(Accel_Y) < VDR.MinAccelY);
    | 
    | % Velocity sensor is zero
    | 
    | aVarTruthTableCondition_4 = logical(abs(Speed) < VDR.MinVelocity);
    | 
    | if (aVarTruthTableCondition_1 && aVarTruthTableCondition_2 && aVarTruthTableCondition_3 && aVarTruthTableCondition_4)
    |     aFcnTruthTableAction_1();
    | else % Default
    |     aFcnTruthTableAction_2();
    | end
    | 
    | function aFcnTruthTableAction_1()
    | 
    | % The car is stationary and can now be started up.
    | 
    | StartUpTest = VDR.PASS;
    | 
    | function aFcnTruthTableAction_2()
    | 
    | % The car sensors readins are incorrect or the car is moving. So the car should not be started up.
    | 
    | StartUpTest = VDR.FAIL;
  function CheckingSensorsTable:
    | function CheckingSensorsTable
    | 
    | aVarTruthTableCondition_1 = false;
    | aVarTruthTableCondition_2 = false;
    | aVarTruthTableCondition_3 = false;
    | aVarTruthTableCondition_4 = false;
    | 
    | 
    | % System Command Torque Check
    | 
    | aVarTruthTableCondition_1 = logical(abs(SystemTrqCmd) > 90);
    | 
    | % APPS competition requirements
    | 
    | aVarTruthTableCondition_2 = logical(abs(APPS1 - APPS2)/APPS1 >= 0.1);
    | 
    | % Accelerator-x sanity check
    | 
    | aVarTruthTableCondition_3 = logical(abs(Accel_X) > VDR.MaxAccelX);
    | 
    | % Accelerator-y sanity check
    | 
    | aVarTruthTableCondition_4 = logical(abs(Accel_Y) > VDR.MaxAccelY);
    | 
    | if (aVarTruthTableCondition_1)
    |     aFcnTruthTableAction_1();
    | elseif (aVarTruthTableCondition_2)
    |     aFcnTruthTableAction_1();
    |     aFcnTruthTableAction_2();
    | elseif (aVarTruthTableCondition_3)
    |     aFcnTruthTableAction_1();
    | elseif (aVarTruthTableCondition_4)
    |     aFcnTruthTableAction_1();
    | else % Default
    |     aFcnTruthTableAction_3();
    | end
    | 
    | function aFcnTruthTableAction_1()
    | 
    | % Impossible and/or out of range values. Must shutdown the vehicle.
    | 
    | SensorFailure = 1;
    | 
    | function aFcnTruthTableAction_2()
    | 
    | % APPS Failure
    | 
    | APPS_Status = VDR.ERROR.APPS.FAILURE;
    | 
    | function aFcnTruthTableAction_3()
    | 
    | % DO NOTHING
  function StartUpTestFnc:
    | function StartUpTestFnc
    | temp = true;
    | if(APPS >= 0 && APPS <= 100)
    |     temp = false;
    | end
    | end
